simulink model "Model5"  (R2020a)
settings: Solver=VariableStepAuto  StartTime=0.0  StopTime=10.0  RelTol=1e-3
undefined symbols (not defined in the file): C, R
settings Model: Creator=HP  LastModifiedBy=HP

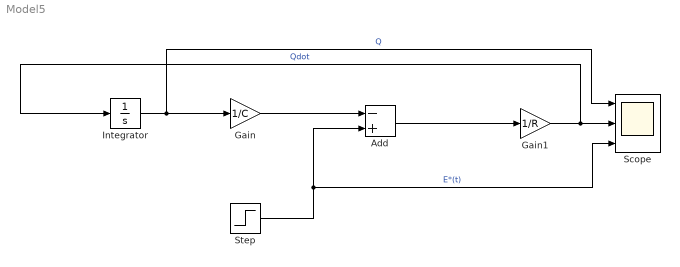
== system Model5 ==
  Add : Sum  Inputs=-+
  Gain : Gain  Gain=1/C
  Gain1 : Gain  Gain=1/R
  Integrator : Integrator
  Scope : Scope  NumInputPorts=3
  Step : Step  SampleTime=0
  wires:
  Integrator/1 -> Scope/1, Gain/1  "Q"
  Gain/1 -> Add/1
  Step/1 -> Add/2, Scope/3  "E*(t)"
  Add/1 -> Gain1/1
  Gain1/1 -> Integrator/1, Scope/2  "Qdot"
